simulink model "Spwm_inverter_motor_drive3"  (R2017a)
settings: Solver=VariableStepAuto  StartTime=0.0  StopTime=3  MaxStep=1e-4  RelTol=1e-3
libraries: powerlib x12, simulink x4, powerlib_meascontrol x3, dspstat3 x2
settings Model: Creator=Halil TEPEDELEN  LastModifiedBy=Halil TEPEDELEN

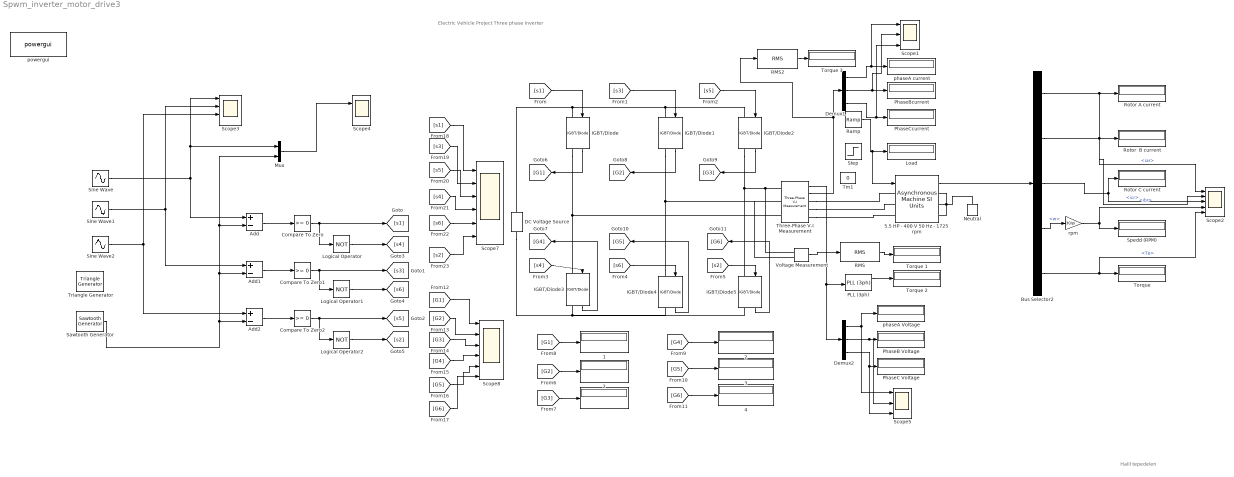
== system Spwm_inverter_motor_drive3 ==
  note: Halil tepedelen
  note: Electric Vehicle Project Three phase inverter
   {,1..2,2..4} (6 alike) : Display
  " Rotor  B current " : Display
  " Rotor A current " : Display
  5.5 HP - 400 V 50 Hz - 1725 rpm : powerlib/Machines/Asynchronous Machine SI Units  RotorType=Wound  PresetModel=No  MechanicalLoad=Torque Tm  ShowDetailedParameters=on  ReferenceFrame=Rotor  Units=SI  MeasurementBus=on  NominalParameters=[4000 200 50]  Stator=[1.405 0.005839]  Rotor=[1.395 0.005839]  Cage1=[ 0.022 0.226/377]  Cage2=[ 0.022 0.226/377]  Lm=0.1722  Mechanical=[0.0131 0.002985 2]  PolePairs=2  InitialConditions="[ 1,0   0,0,0   0,0,0 ]"  SimulateSaturation=off  Saturation=[14.03593122, 27.81365428, 53.79336849, 72.68890987, 97.98006896, 148.6815601, 215.7428561, 302.9841135, 420.4778367 ; 230, 322, 414, 460, 506, 552, 598, 644, 690]  LoadFlowParameters=1492000  TsPowergui=0  TsBlock=-1  IterativeModel=Trapezoidal non iterative  IterativeDiscreteModel=Trapezoidal non iterative  Pmec=4000
  Add : Sum  Inputs=+-
  Add1 : Sum  Inputs=+-
  Add2 : Sum  Inputs=+-
  Bus Selector2 : BusSelector  OutputSignals=iar,ibr,icr,w,Te
  Compare To Zero : simulink/Logic and Bit Operations/Compare To Zero  relop=>=  OutDataTypeStr=boolean
  Compare To Zero1 : simulink/Logic and Bit Operations/Compare To Zero  relop=>=  OutDataTypeStr=boolean
  Compare To Zero2 : simulink/Logic and Bit Operations/Compare To Zero  relop=>=  OutDataTypeStr=boolean
  DC Voltage Source : powerlib/Electrical Sources/DC Voltage Source  Amplitude=200  Measurements=Voltage
  Demux1 : Demux  Outputs=3
  Demux2 : Demux  Outputs=3
  IGBT/Diode{,1..5} (6 alike) : powerlib/Power Electronics/IGBT//Diode  Ron=1e-3  Rs=1e5  Cs=inf  Measurements=on
  Load : Display
  Logical Operator : Logic  Operator=NOT  AllPortsSameDT=off  OutDataTypeStr=boolean
  Logical Operator1 : Logic  Operator=NOT  AllPortsSameDT=off  OutDataTypeStr=boolean
  Logical Operator2 : Logic  Operator=NOT  AllPortsSameDT=off  OutDataTypeStr=boolean
  Mux : Mux  Inputs=2
  Neutral : powerlib/Elements/Neutral  LConnTagsString=a  NodeNumber=10
      settings: SourceProductName=Simscape Power Systems  SourceProductBaseCode=PS
  PLL (3ph) : powerlib_meascontrol/PLL/PLL (3ph)  Fmin=45  Par_Init=[0, 60]  ParK=[180, 3200, 1]  TcD=1e-4  MaxRateChangeFreq=12  FilterCutOffFreq=25  Ts=0  AGC=on
  PhaseB Voltage : Display
  PhaseBcurrent : Display
  PhaseC Voltage : Display
  PhaseCcurrent : Display
  RMS : dspstat3/RMS  run=off  directionMode=Each column  dimension=1  InputProcessing=Columns as channels (frame based)  reset_popup=None
  RMS2 : dspstat3/RMS  run=off  directionMode=Each column  dimension=1  InputProcessing=Columns as channels (frame based)  reset_popup=None
  Ramp : simulink/Sources/Ramp  slope=30  start=0  X0=1
  "Rotor C current " : Display
  Sawtooth Generator : powerlib_meascontrol/Pulse & Signal Generators/Sawtooth Generator  Freq=1e3  Phase=180  Ts=0
      settings: SourceProductName=Simscape Power Systems
  Scope1 : Scope  NumInputPorts=3
  Scope2 : Scope  NumInputPorts=5
  Scope3 : Scope  NumInputPorts=4
  Scope4 : Scope  NumInputPorts=2
  Scope5 : Scope  NumInputPorts=3
  Scope7 : Scope  NumInputPorts=6
  Scope8 : Scope  NumInputPorts=6
  Sine Wave : Sin  Frequency=2*pi*50  SampleTime=0
  Sine Wave1 : Sin  Frequency=2*pi*50  Phase=2*pi/3  SampleTime=0
  Sine Wave2 : Sin  Frequency=2*pi*50  Phase=-2*pi/3  SampleTime=0
  "Spedd (RPM) " : Display
  Step : Step  Time=0.13  Before=3  After=38  SampleTime=0.1  VectorParams1D=off
  Three-Phase V-I Measurement : powerlib/Measurements/Three-Phase V-I Measurement  VoltageMeasurement=phase-to-phase  SetLabelV=off  LabelV=Vabc  Vpu=off  VpuLL=off  CurrentMeasurement=yes  SetLabelI=off  LabelI=Iabc  Ipu=off  Pbase=100e6  Vbase=500e3  OutputType=Complex  PhasorSimulation=off  PSBequivalent=0
  Tm1 : Constant  Value=0
  Torque {,1..3} (4 alike) : Display
  Triangle Generator : powerlib_meascontrol/Pulse & Signal Generators/Triangle Generator  Freq=1e3  Phase=90  Ts=0
  Voltage Measurement : powerlib/Measurements/Voltage Measurement  PhasorSimulation=off  OutputType=Complex  PSBequivalent=0
  phaseA Voltage : Display
  phaseA current : Display
  powergui : powerlib/powergui  Priority=1  SimulationMode=Continuous  SampleTime=50e-6  frequency=60  Iterations=50  frequencyindice=0  Pbase=100e6  ErrMax=1e-4  UnitsV=kV  UnitsW=MW  buscounter=0  FunctionMessages=off  echomessages=off  EnableUseOfTLC=off  CurrentSourceSwitches=off  DisableSnubberDevices=off  DisableRonSwitches=off  DisableVfSwitches=off  DisplayEquations=off  SolverType=Tustin/Backward Euler (TBE)  Interpol=off  ExternalGateDelay=off  methode=off  Ts=100  x0status=blocks  SPID=on  SwTol=0  HookPort=off  RestoreLinks=warning  ResistiveCurrentMeasurement=off  Frange=[0:2:500]  Ylog=off  Xlog=on  ShowGrid=off  save=off  variable=ZData  structure=0  ZoomFFT=off  StartTime=0.0  cycles=1  DisplayStyle=1  fundamental=60  FreqAxis=off  MaxFrequency=1000  frequencyindicesteady=1  RmsSteady=1  display=off
  rpm : Gain  Gain=30/pi  SaturateOnIntegerOverflow=on  OutDataTypeStr=Inherit: Same as input  ParamDataTypeStr=Inherit: Same as input
  wires:
  Sine Wave1/1 -> Add1/1, Scope3/2
  Sine Wave/1 -> Scope3/1, Mux/1, Add/1
  Sine Wave2/1 -> Scope3/3, Add2/1
  Add/1 -> Compare To Zero/1
  Add1/1 -> Compare To Zero1/1
  Add2/1 -> Compare To Zero2/1
  Mux/1 -> Scope4/1
  Compare To Zero/1 -> Logical Operator/1, [s1]
  Compare To Zero2/1 -> Logical Operator2/1, [s5]
  Compare To Zero1/1 -> Logical Operator1/1, [s3]
  Logical Operator/1 -> [s4]
  Logical Operator1/1 -> [s6]
  Logical Operator2/1 -> [s2]
  Three-Phase V-I Measurement/2 -> RMS2/1, Demux1/1
  Demux1/3 -> Scope1/3, PhaseCcurrent/1
  Demux1/1 -> Scope1/1, phaseA current/1
  5.5 HP - 400 V 50 Hz - 1725 rpm/1 -> Bus Selector2/1
  Bus Selector2/1 -> Scope2/1, " Rotor A current "/1  "<iar>"
  Bus Selector2/2 -> Scope2/2, " Rotor  B current "/1  "<ibr>"
  Bus Selector2/3 -> "Rotor C current "/1, Scope2/3  "<icr>"
  Bus Selector2/5 -> Scope2/5, "Torque "/1  "<Te>"
  Demux2/1 -> Scope5/1, phaseA Voltage/1
  Demux2/2 -> Scope5/2, PhaseB Voltage/1
  Demux2/3 -> Scope5/3, PhaseC Voltage/1
  Three-Phase V-I Measurement/1 -> PLL (3ph)/1, Demux2/1
  [G1] -> " 1"/1
  [G2] -> " 2"/1
  [G3] -> " "/1
  [G4] -> " 2"/1
  [G5] -> " 3"/1
  [G6] -> " 4"/1
  [G1] -> Scope8/1
  [G2] -> Scope8/2
  [G3] -> Scope8/3
  [G4] -> Scope8/4
  [G5] -> Scope8/5
  [G6] -> Scope8/6
  [s1] -> Scope7/1
  [s3] -> Scope7/2
  [s5] -> Scope7/3
  [s4] -> Scope7/4
  [s6] -> Scope7/5
  [s2] -> Scope7/6
  Bus Selector2/4 -> rpm/1  "<w>"
  rpm/1 -> "Spedd (RPM) "/1, Scope2/4
  IGBT/Diode/1 -> [G1]
  IGBT/Diode1/1 -> [G2]
  IGBT/Diode3/1 -> [G4]
  IGBT/Diode4/1 -> [G5]
  IGBT/Diode5/1 -> [G6]
  IGBT/Diode2/1 -> [G3]
  [s5] -> IGBT/Diode2/1
  [s3] -> IGBT/Diode1/1
  [s1] -> IGBT/Diode/1
  [s2] -> IGBT/Diode5/1
  [s6] -> IGBT/Diode4/1
  [s4] -> IGBT/Diode3/1
  Voltage Measurement/1 -> RMS/1
  RMS/1 -> Torque 1/1
  PLL (3ph)/1 -> Torque 2/1
  RMS2/1 -> Torque 3/1
  Demux1/2 -> Scope1/2, PhaseBcurrent/1
  Sawtooth Generator/1 -> Add2/2, Mux/2, Add/2, Add1/2
  Ramp/1 -> 5.5 HP - 400 V 50 Hz - 1725 rpm/1, Load/1
  connections:
  Three-Phase V-I Measurement/RConn1 -- 5.5 HP - 400 V 50 Hz - 1725 rpm/LConn1
  Three-Phase V-I Measurement/RConn2 -- 5.5 HP - 400 V 50 Hz - 1725 rpm/LConn2
  Three-Phase V-I Measurement/RConn3 -- 5.5 HP - 400 V 50 Hz - 1725 rpm/LConn3
  DC Voltage Source/RConn1 -- IGBT/Diode/LConn1 -- IGBT/Diode1/LConn1 -- IGBT/Diode2/LConn1
  IGBT/Diode/RConn1 -- Three-Phase V-I Measurement/LConn3 -- IGBT/Diode3/LConn1
  IGBT/Diode1/RConn1 -- Voltage Measurement/LConn2 -- Three-Phase V-I Measurement/LConn2 -- IGBT/Diode4/LConn1
  IGBT/Diode2/RConn1 -- IGBT/Diode5/LConn1 -- Voltage Measurement/LConn1 -- Three-Phase V-I Measurement/LConn1
  DC Voltage Source/LConn1 -- IGBT/Diode4/RConn1 -- IGBT/Diode5/RConn1 -- IGBT/Diode3/RConn1
  5.5 HP - 400 V 50 Hz - 1725 rpm/RConn1 -- Neutral/LConn1 -- 5.5 HP - 400 V 50 Hz - 1725 rpm/RConn3 -- 5.5 HP - 400 V 50 Hz - 1725 rpm/RConn2
